simulink model "ddrxpose_21a_generic"  (R2021a)
settings: Solver=VariableStepAuto  StartTime=0.0  StopTime=300e-6  FixedStep=Ts  RelTol=1e-3  EnableMultiTasking=on
InitFcn:
  | model_init_sim;
model workspace (MAT data in the model file):
  mwTaskManagerKernelLatency = 0
  socvcb = containers.Map
  socvcb.serialization.keys = {74.0001220703, 74.0092773438, 74.0178222656, 75.0001220703, 75.0092773438, 75.0178222656}
  socvcb.serialization.values : function handle (value not decoded)
  socvcb.serialization.uniformity = 0
  socvcb.serialization.keyType = 'double'
  socvcb.serialization.valueType = 'any'
values from neighbouring files (symbols this model uses):
  hBlank = 20    [model_init_sim.m]
  inputImageDDROffset = uint32(hex2dec('00000000'))    [model_init_sim.m]
  MatrixInput = reshape(MatrixInputArr,[N1,N2])    [matrix_init.m]
  pAXIDataWidthBytes = 4    [model_init_sim.m]
  pMaxBankLines = 6    [model_init_sim.m]
  pMaxNumBanks = 3    [model_init_sim.m]
  pNumCols = 30    [model_init_sim.m]
  pNumRows = 30    [model_init_sim.m]
  Ts = 1/(totalPixels*60)    [model_init_sim.m]
libraries: socmemlib x2, hdlsllib x2, simulink x1
settings Model: DataTypeOverride=Off  SimulationMode=accelerator  ExtModeTrigDuration=1  Creator=skuznick  LastModifiedBy=darenlee
settings SolverCC: AlgebraicLoopSolver=TrustRegion  PositivePriorityOrder=on
settings DataIOCC: LimitDataPoints=on  SaveOutput=off  DSMLogging=off  InspectSignalLogs=on  VisualizeSimOutput=off  SaveTime=off
settings OptimizationCC: BlockReduction=off  ConditionallyExecuteInputs=off  DefaultUnderspecifiedDataType=single  EnhancedBackFolding=on  PassReuseOutputArgsAs=Individual arguments  ZeroExternalMemoryAtStartup=off  ZeroInternalMemoryAtStartup=off  EfficientFloat2IntCast=on  MaxStackSize=64  SimCompilerOptimization=on  OptimizeBlockOrder=speed  DifferentSizesBufferReuse=on  OptimizationCustomize=off  EfficientTunableParamExpr=on
settings DebuggingCC: AlgebraicLoopMsg=error  SingleTaskRateTransMsg=error  ParameterPrecisionLossMsg=none  ParameterTunabilityLossMsg=error  AllowSymbolicDim=off  PregeneratedLibrarySubsystemCodeDiagnostic=none  SFUnexpectedBacktrackingDiag=warning  SFNoUnconditionalDefaultTransitionDiag=warning  SFExecutionAtInitializationDiag=none  SFMachineParentedDataDiag=warning  IntegerSaturationMsg=none  ArithmeticOperatorsInVariantConditions=warning
settings HardwareCC: ProdBitPerLong=64  ProdLargestAtomicInteger=LongLong  ProdLargestAtomicFloat=Double  ProdLongLongMode=on  ProdHWDeviceType=ARM Compatible->ARM 64-bit (LP64)  ProdEqTarget=off  HardwareBoardFeatureSet=SoCBlockset
settings SFSimCC: SimUseLocalCustomCode=off  MATLABDynamicMemAlloc=off  CustomCodeUndefinedFunction=UseInterfaceOnly
settings RTWCC: SystemTargetFile=ert.tlc  HardwareBoard=Xilinx Zynq UltraScale+ MPSoC ZCU102 Evaluation Kit  TLCOptions="-aInlineSetEventsForThisBaseRateFcn=TLC_FALSE -aSuppressMultiTaskScheduler=TLC_FALSE  -aRateBasedStepFcn=0"  TemplateMakefile=ert_default_tmf  GenerateReport=on  RTWUseLocalCustomCode=off  Toolchain=Linaro AArch64 Linux v6.3.1  BuildConfiguration=Faster Runs  IncludeHyperlinkInReport=on  LaunchReport=on  GenerateTraceInfo=on  GenerateTraceReport=on  GenerateTraceReportSl=on  GenerateTraceReportSf=on  GenerateTraceReportEml=on
settings CodeAppCC: ForceParamTrailComments=on  IgnoreCustomStorageClasses=off  OperatorAnnotations=on  SimulinkDataObjDesc=on  SFDataObjDesc=on  InsertBlockDesc=on
settings ConfigComp: CovMetricSettings=dw  CovSaveCumulativeToWorkspaceVar=on  CovSaveSingleToWorkspaceVar=on  CovExternalEMLEnable=off  CovSFcnEnable=off

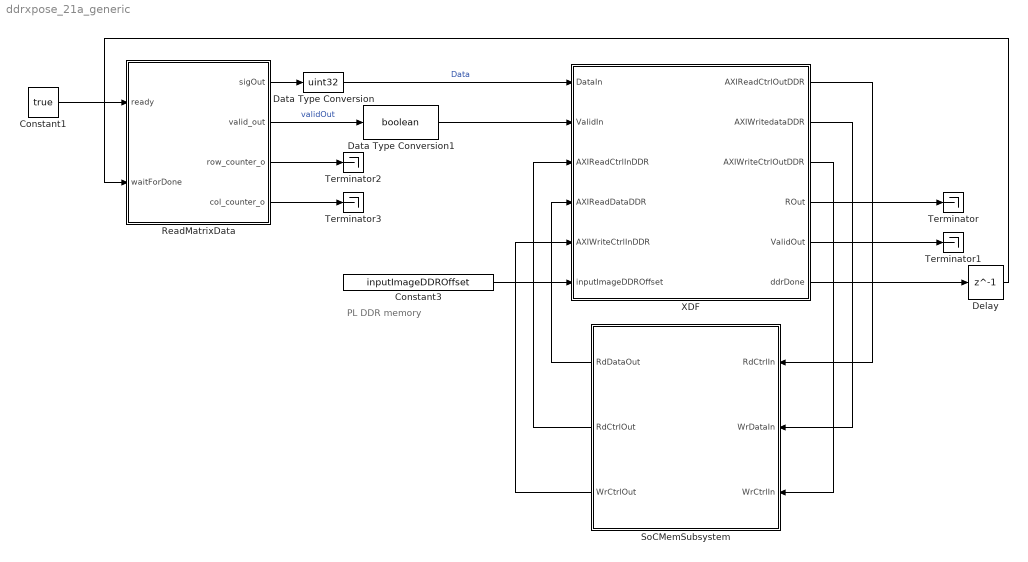
== system ddrxpose_21a_generic ==
  note: PL DDR memory
  Constant1 : Constant  Value=true  SampleTime=-1
  Constant3 : Constant  Value=inputImageDDROffset  OutDataTypeStr=uint32  SampleTime=-1
  Data Type Conversion : DataTypeConversion  OutDataTypeStr=uint32
  Data Type Conversion1 : DataTypeConversion  OutDataTypeStr=boolean
  Delay : Delay  DelayLength=1
  ReadMatrixData : MATLAB Function  TreatAsAtomicUnit=on  SystemSampleTime=Ts  mask{MatrixInput=MatrixInput, ValidGap=16*3 % 48 clock cycles, Ts=Ts}
      mask prompts: MatrixInput "Matrix value"; ValidGap "Valid Gap between columns"; Ts "Sample Time"
  SoCMemSubsystem : Subsystem
  Terminator{,1..3} (4 alike) : Terminator
  XDF : Subsystem  TreatAsAtomicUnit=on
  wires:
  SoCMemSubsystem/2(RdCtrlOut) -> XDF/3(AXIReadCtrlInDDR)
  SoCMemSubsystem/3(WrCtrlOut) -> XDF/5(AXIWriteCtrlInDDR)
  SoCMemSubsystem/1(RdDataOut) -> XDF/4(AXIReadDataDDR)
  XDF/1(AXIReadCtrlOutDDR) -> SoCMemSubsystem/1(RdCtrlIn)
  XDF/2(AXIWritedataDDR) -> SoCMemSubsystem/2(WrDataIn)
  XDF/3(AXIWriteCtrlOutDDR) -> SoCMemSubsystem/3(WrCtrlIn)
  Constant3/1 -> XDF/6(inputImageDDROffset)
  XDF/6(ddrDone) -> Delay/1
  Constant1/1 -> ReadMatrixData/1(ready)
  ReadMatrixData/1(sigOut) -> Data Type Conversion/1
  ReadMatrixData/2(valid_out) -> Data Type Conversion1/1  "validOut"
  ReadMatrixData/3(row_counter_o) -> Terminator2/1
  ReadMatrixData/4(col_counter_o) -> Terminator3/1
  Data Type Conversion/1 -> XDF/1(DataIn)  "Data"
  Delay/1 -> ReadMatrixData/2(waitForDone)
  XDF/4(ROut) -> Terminator/1
  XDF/5(ValidOut) -> Terminator1/1
  Data Type Conversion1/1 -> XDF/2(ValidIn)

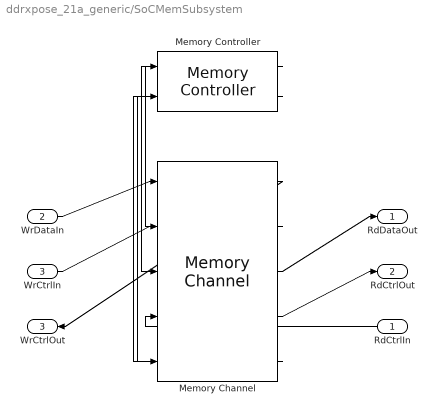
== system ddrxpose_21a_generic/SoCMemSubsystem ==
  RdCtrlIn : Inport
  WrDataIn : Inport  Port=2
  WrCtrlIn : Inport  Port=3
  Memory Channel : socmemlib/Memory Channel  InstantiateOnLoad=on  ChannelType=AXI4 Random Access  MRBufferSize=pNumCols*pNumRows*4*4  MRNumBuffers=1  BurstLengthWriterChIf=256  BurstLengthReaderChIf=256  UseValuesFromTargetHardwareResources=off  ReaderWriterUseSameValues=on  FIFODepthWriter=8  FIFODepthReader=8  FIFOAFullDepthWriter=6  FIFOAFullDepthReader=6  ICClockFrequencyWriter=300  ICClockFrequencyReader=300  ICDataWidthWriter=32  ICDataWidthReader=32  ChDimensionsWriterChIf=1  ChTypeWriterChIf=fixdt(0,(pAXIDataWidthBytes*8),0)  ChFrameSampleTimeWriterChIf=Ts  ChBitPackedWriterChIf=off  OutSigSpecMatchesInSigSpec=on  ChDimensionsReaderChIf=1  ChTypeWithInhReaderChIf=uint8  ChFrameSampleTimeReaderChIf=6.734006734006734e-09  ChBitPackedReaderChIf=off  InsertInactivePixelClocksReaderChIf=off  FrameSizeReaderChIf=160x120p  ProtocolWriter=AXI4  ProtocolReader=AXI4  ChTypeReaderChIf=fixdt(0,32,0)  LastTargetBoard=Xilinx Zynq UltraScale+ MPSoC ZCU102 Evaluation Kit  Beta2Compatible=off  MRRegionSize=14400  DiagnosticLevel=Basic diagnostic signals  MRBaseAddress=hex2dec('00010000')  UseTargetGlobalValues=off  InterruptHandlingTimeWriterChIf=10e-6  BufferEventIDWriterChIf=NOT_USED  BufferLengthReaderChIf=NOT_USED  InterruptHandlingTimeReaderChIf=10e-6  BufferEventIDReaderChIf=NOT_USED
      settings: SourceProductBaseCode=HW
  Memory Controller : socmemlib/Memory Controller  InstantiateOnLoad=on  NumMasters=2  ICArbitrationPolicy=Round robin  UseValuesFromTargetHardwareResources=off  ControllerFrequency=300  ControllerDataWidth=128  BandwidthDerating=2.3  WriteFirstTransferLatency=19  ReadFirstTransferLatency=2  WriteLastTransferLatency=4  ReadLastTransferLatency=1  LastTargetBoard=Xilinx Zynq UltraScale+ MPSoC ZCU102 Evaluation Kit  DiagnosticLevel=Basic diagnostic signals.2  MAX_NUM_MASTERS=12  DDRRefreshLength=4  DDRRefreshInterval=7.8  PlotTimeResolution=100e-6
      settings: SourceProductBaseCode=HW
  RdDataOut : Outport  VectorParamsAs1DForOutWhenUnconnected=off
  RdCtrlOut : Outport  Port=2  VectorParamsAs1DForOutWhenUnconnected=off
  WrCtrlOut : Outport  Port=3  VectorParamsAs1DForOutWhenUnconnected=off
  wires:
  Memory Channel/3 -> RdDataOut/1
  Memory Channel/4 -> RdCtrlOut/1
  Memory Channel/1 -> WrCtrlOut/1
  RdCtrlIn/1 -> Memory Channel/4
  WrDataIn/1 -> Memory Channel/1
  WrCtrlIn/1 -> Memory Channel/2
  Memory Channel/2 -> Memory Controller/1
  Memory Controller/1 -> Memory Channel/3
  Memory Controller/2 -> Memory Channel/5
  Memory Channel/5 -> Memory Controller/2

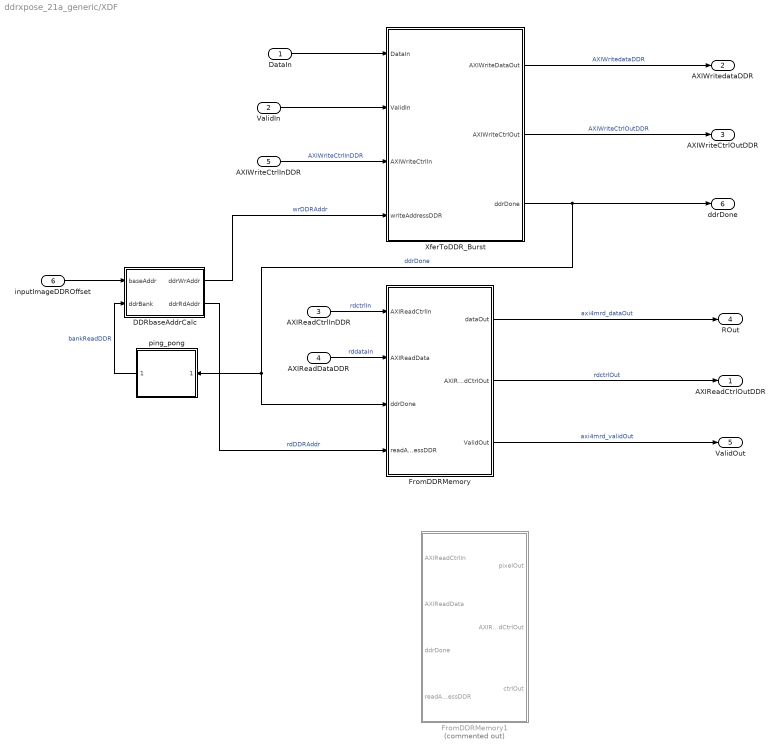
== system ddrxpose_21a_generic/XDF ==
  DataIn : Inport
  ValidIn : Inport  Port=2
  AXIReadCtrlInDDR : Inport  Port=3
  AXIReadDataDDR : Inport  Port=4
  AXIWriteCtrlInDDR : Inport  Port=5
  inputImageDDROffset : Inport  Port=6
  DDRbaseAddrCalc : Subsystem
  FromDDRMemory : Subsystem
  FromDDRMemory1 : Subsystem  Commented=on
  XferToDDR_Burst : Subsystem  VariantControl=XferToDDR_Burst
  ping_pong : Subsystem
  AXIReadCtrlOutDDR : Outport  VectorParamsAs1DForOutWhenUnconnected=off
  AXIWritedataDDR : Outport  Port=2  VectorParamsAs1DForOutWhenUnconnected=off
  AXIWriteCtrlOutDDR : Outport  Port=3  VectorParamsAs1DForOutWhenUnconnected=off
  ROut : Outport  Port=4  VectorParamsAs1DForOutWhenUnconnected=off
  ValidOut : Outport  Port=5
  ddrDone : Outport  Port=6
  wires:
  AXIWriteCtrlInDDR/1 -> XferToDDR_Burst/3(AXIWriteCtrlIn)  "AXIWriteCtrlInDDR"
  XferToDDR_Burst/1(AXIWriteDataOut) -> AXIWritedataDDR/1  "AXIWritedataDDR"
  XferToDDR_Burst/2(AXIWriteCtrlOut) -> AXIWriteCtrlOutDDR/1  "AXIWriteCtrlOutDDR"
  AXIReadCtrlInDDR/1 -> FromDDRMemory/1(AXIReadCtrlIn)  "rdctrlIn"
  AXIReadDataDDR/1 -> FromDDRMemory/2(AXIReadData)  "rddataIn"
  XferToDDR_Burst/3(ddrDone) -> ping_pong/1(ddrDone), FromDDRMemory/3(ddrDone), ddrDone/1  "ddrDone"
  FromDDRMemory/1(dataOut) -> ROut/1  "axi4mrd_dataOut"
  FromDDRMemory/2(AXIReadCtrlOut) -> AXIReadCtrlOutDDR/1  "rdctrlOut"
  DDRbaseAddrCalc/1(ddrWrAddr) -> XferToDDR_Burst/4(writeAddressDDR)  "wrDDRAddr"
  inputImageDDROffset/1 -> DDRbaseAddrCalc/1(baseAddr)
  ping_pong/1(ddrBank) -> DDRbaseAddrCalc/2(ddrBank)  "bankReadDDR"
  DDRbaseAddrCalc/2(ddrRdAddr) -> FromDDRMemory/4(readAddressDDR)  "rdDDRAddr"
  DataIn/1 -> XferToDDR_Burst/1(DataIn)
  ValidIn/1 -> XferToDDR_Burst/2(ValidIn)
  FromDDRMemory/3(ValidOut) -> ValidOut/1  "axi4mrd_validOut"

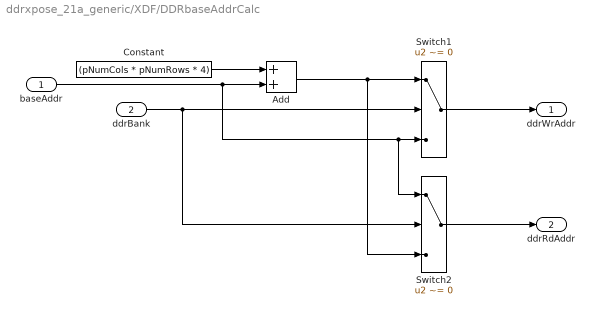
== system ddrxpose_21a_generic/XDF/DDRbaseAddrCalc ==
  baseAddr : Inport
  ddrBank : Inport  Port=2
  Add : Sum  OutDataTypeStr=uint32
  Constant : Constant  Value=(pNumCols * pNumRows * 4)  OutDataTypeStr=uint32  SampleTime=-1
  Switch1 : Switch  Criteria=u2 ~= 0
  Switch2 : Switch  Criteria=u2 ~= 0
  ddrWrAddr : Outport
  ddrRdAddr : Outport  Port=2
  wires:
  Constant/1 -> Add/1
  Add/1 -> Switch2/3, Switch1/1
  Switch1/1 -> ddrWrAddr/1
  ddrBank/1 -> Switch2/2, Switch1/2
  baseAddr/1 -> Switch2/1, Switch1/3, Add/2
  Switch2/1 -> ddrRdAddr/1

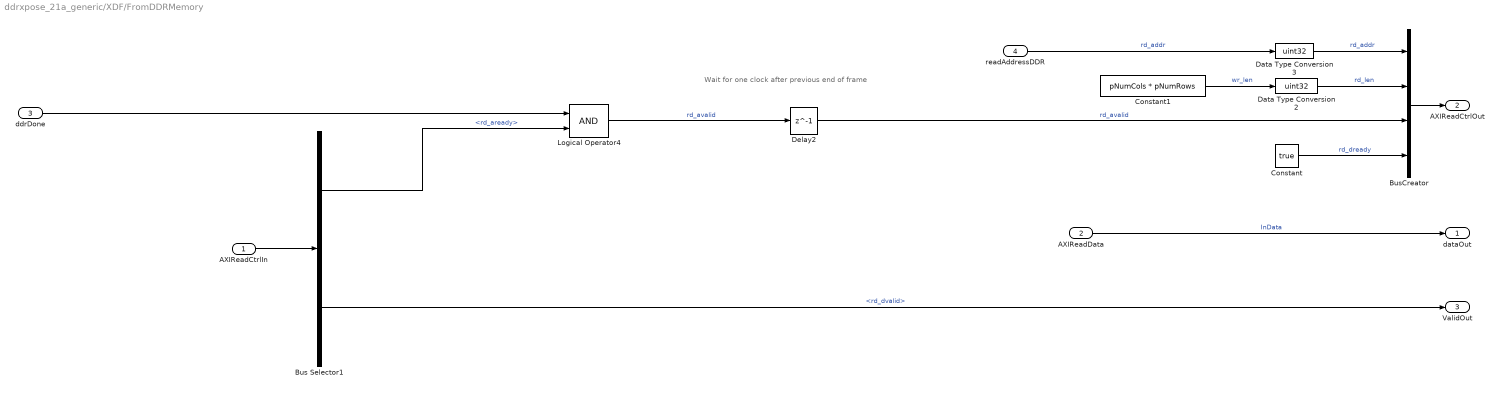
== system ddrxpose_21a_generic/XDF/FromDDRMemory ==
  note: Wait for one clock after previous end of frame
  AXIReadCtrlIn : Inport
  AXIReadData : Inport  Port=2
  ddrDone : Inport  Port=3
  readAddressDDR : Inport  Port=4
  Bus Selector1 : BusSelector  OutputSignals=rd_aready,rd_dvalid
  BusCreator : BusCreator  Inputs=4
  Constant : Constant  Value=true  SampleTime=-1
  Constant1 : Constant  Value=pNumCols * pNumRows  OutDataTypeStr=uint32  SampleTime=-1
  Data Type Conversion2 : DataTypeConversion  OutDataTypeStr=uint32
  Data Type Conversion3 : DataTypeConversion  OutDataTypeStr=uint32
  Delay2 : Delay  DelayLength=1  InitialCondition=0
  Logical Operator4 : Logic  IconShape=distinctive  AllPortsSameDT=off  OutDataTypeStr=boolean
  dataOut : Outport  VectorParamsAs1DForOutWhenUnconnected=off
  AXIReadCtrlOut : Outport  Port=2  VectorParamsAs1DForOutWhenUnconnected=off
  ValidOut : Outport  Port=3
  wires:
  Delay2/1 -> BusCreator/3  "rd_avalid"
  Constant/1 -> BusCreator/4  "rd_dready"
  Bus Selector1/1 -> Logical Operator4/2  "<rd_aready>"
  BusCreator/1 -> AXIReadCtrlOut/1
  Bus Selector1/2 -> ValidOut/1  "<rd_dvalid>"
  Logical Operator4/1 -> Delay2/1  "rd_avalid"
  AXIReadData/1 -> dataOut/1  "InData"
  Constant1/1 -> Data Type Conversion2/1  "wr_len"
  Data Type Conversion2/1 -> BusCreator/2  "rd_len"
  AXIReadCtrlIn/1 -> Bus Selector1/1
  Data Type Conversion3/1 -> BusCreator/1  "rd_addr"
  readAddressDDR/1 -> Data Type Conversion3/1  "rd_addr"
  ddrDone/1 -> Logical Operator4/1

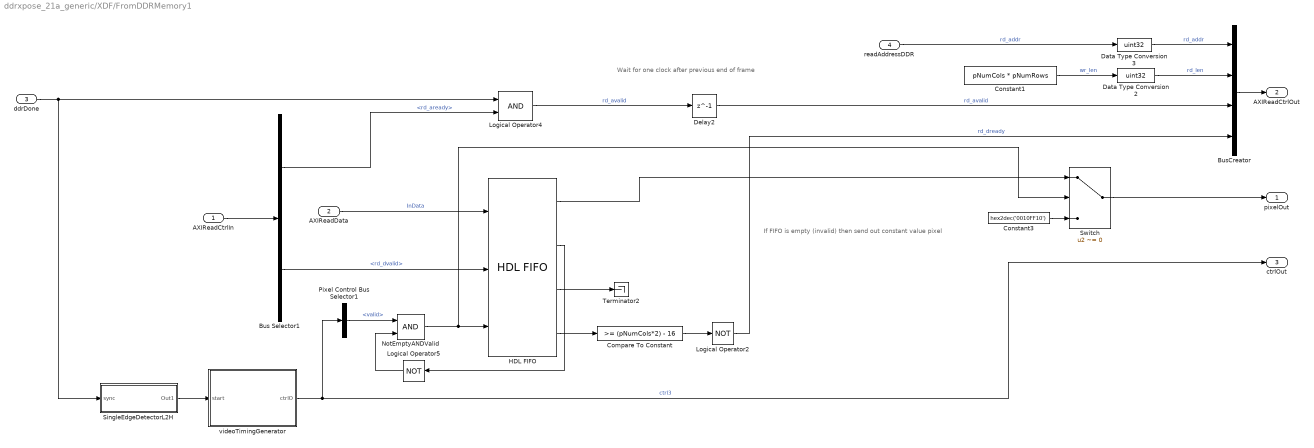
== system ddrxpose_21a_generic/XDF/FromDDRMemory1 ==
  note: Wait for one clock after previous end of frame
  note: If FIFO is empty (invalid) then send out constant value pixel
  AXIReadCtrlIn : Inport
  AXIReadData : Inport  Port=2
  ddrDone : Inport  Port=3
  readAddressDDR : Inport  Port=4
  Bus Selector1 : BusSelector  OutputSignals=rd_aready,rd_dvalid
  BusCreator : BusCreator  Inputs=4
  Compare To Constant : simulink/Logic and Bit Operations/Compare To Constant  relop=>=  const=(pNumCols*2) - 16  OutDataTypeStr=boolean
  Constant1 : Constant  Value=pNumCols * pNumRows  OutDataTypeStr=uint32  SampleTime=-1
  Constant3 : Constant  Value=hex2dec('0010FF10')  OutDataTypeStr=fixdt(0,32,0)  SampleTime=-1
  Data Type Conversion2 : DataTypeConversion  OutDataTypeStr=uint32
  Data Type Conversion3 : DataTypeConversion  OutDataTypeStr=uint32
  Delay2 : Delay  DelayLength=1  InitialCondition=0
  HDL FIFO : hdlsllib/HDL RAMs/HDL FIFO  fifo_size=pNumCols*2  mode=FWFT  ratio=1  push_msg=Warning  pop_msg=Warning  show_empty=on  show_full=on  show_num=on  LabelModeActiveChoice_Mode=FWFT
      settings: SourceProductBaseCode=SL
  Logical Operator2 : Logic  Operator=NOT  IconShape=distinctive  AllPortsSameDT=off  OutDataTypeStr=boolean
  Logical Operator4 : Logic  IconShape=distinctive  AllPortsSameDT=off  OutDataTypeStr=boolean
  Logical Operator5 : Logic  Operator=NOT  IconShape=distinctive  AllPortsSameDT=off  OutDataTypeStr=boolean
  NotEmptyANDValid : Logic  IconShape=distinctive  AllPortsSameDT=off  OutDataTypeStr=boolean
  Pixel Control Bus Selector1 : BusSelector  OutputSignals=valid
  SingleEdgeDetectorL2H : Subsystem  TreatAsAtomicUnit=on
  Switch : Switch  Criteria=u2 ~= 0
  Terminator2 : Terminator
  videoTimingGenerator : MATLAB Function  TreatAsAtomicUnit=on  VariantControl=Variant2  mask{hSize=pNumCols, vSize=pNumRows, hBlank=hBlank, vBlank=2, delayStartClks=pNumCols*5}
      mask prompts: hSize "Frame Width"; vSize "Frame Height"; hBlank "Horz Blanking"; vBlank "Vert Blanking"; delayStartClks "Start Delay in Clocks"
  pixelOut : Outport  VectorParamsAs1DForOutWhenUnconnected=off
  AXIReadCtrlOut : Outport  Port=2  VectorParamsAs1DForOutWhenUnconnected=off
  ctrlOut : Outport  Port=3  VectorParamsAs1DForOutWhenUnconnected=off
  wires:
  Switch/1 -> pixelOut/1
  NotEmptyANDValid/1 -> Switch/2, HDL FIFO/3
  Constant3/1 -> Switch/3
  Delay2/1 -> BusCreator/3  "rd_avalid"
  Logical Operator2/1 -> BusCreator/4  "rd_dready"
  Pixel Control Bus Selector1/1 -> NotEmptyANDValid/1  "<valid>"
  HDL FIFO/1 -> Switch/1
  Bus Selector1/1 -> Logical Operator4/2  "<rd_aready>"
  Logical Operator5/1 -> NotEmptyANDValid/2
  BusCreator/1 -> AXIReadCtrlOut/1
  Bus Selector1/2 -> HDL FIFO/2  "<rd_dvalid>"
  Logical Operator4/1 -> Delay2/1  "rd_avalid"
  HDL FIFO/2 -> Logical Operator5/1
  AXIReadData/1 -> HDL FIFO/1  "InData"
  Constant1/1 -> Data Type Conversion2/1  "wr_len"
  Data Type Conversion2/1 -> BusCreator/2  "rd_len"
  AXIReadCtrlIn/1 -> Bus Selector1/1
  Data Type Conversion3/1 -> BusCreator/1  "rd_addr"
  readAddressDDR/1 -> Data Type Conversion3/1  "rd_addr"
  HDL FIFO/4 -> Compare To Constant/1
  Compare To Constant/1 -> Logical Operator2/1
  HDL FIFO/3 -> Terminator2/1
  videoTimingGenerator/1(ctrlO) -> ctrlOut/1, Pixel Control Bus Selector1/1  "ctrl3"
  ddrDone/1 -> SingleEdgeDetectorL2H/1(sync), Logical Operator4/1
  SingleEdgeDetectorL2H/1(Out1) -> videoTimingGenerator/1(start)

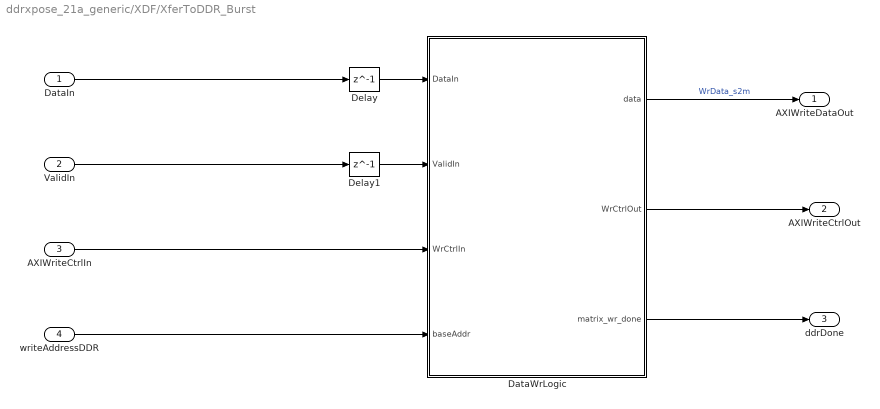
== system ddrxpose_21a_generic/XDF/XferToDDR_Burst ==
  DataIn : Inport
  ValidIn : Inport  Port=2
  AXIWriteCtrlIn : Inport  Port=3
  writeAddressDDR : Inport  Port=4
  DataWrLogic : Subsystem
  Delay : Delay  DelayLength=1
  Delay1 : Delay  DelayLength=1
  AXIWriteDataOut : Outport
  AXIWriteCtrlOut : Outport  Port=2
  ddrDone : Outport  Port=3
  wires:
  Delay1/1 -> DataWrLogic/2(ValidIn)
  Delay/1 -> DataWrLogic/1(DataIn)
  DataWrLogic/1(data) -> AXIWriteDataOut/1  "WrData_s2m"
  DataIn/1 -> Delay/1
  DataWrLogic/2(WrCtrlOut) -> AXIWriteCtrlOut/1
  AXIWriteCtrlIn/1 -> DataWrLogic/3(WrCtrlIn)
  DataWrLogic/3(matrix_wr_done) -> ddrDone/1
  ValidIn/1 -> Delay1/1
  writeAddressDDR/1 -> DataWrLogic/4(baseAddr)

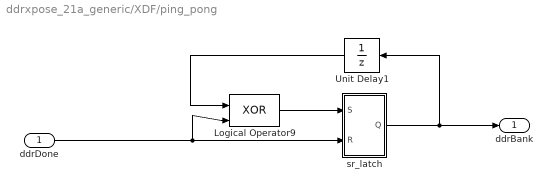
== system ddrxpose_21a_generic/XDF/ping_pong ==
  ddrDone : Inport
  Logical Operator9 : Logic  Operator=XOR  IconShape=distinctive  AllPortsSameDT=off  OutDataTypeStr=boolean
  Unit Delay1 : UnitDelay  SampleTime=-1  HasFrameUpgradeWarning=on
  sr_latch : Subsystem
  ddrBank : Outport  VectorParamsAs1DForOutWhenUnconnected=off
  wires:
  Unit Delay1/1 -> Logical Operator9/1
  Logical Operator9/1 -> sr_latch/1(S)
  ddrDone/1 -> sr_latch/2(R), Logical Operator9/2
  sr_latch/1(Q) -> Unit Delay1/1, ddrBank/1

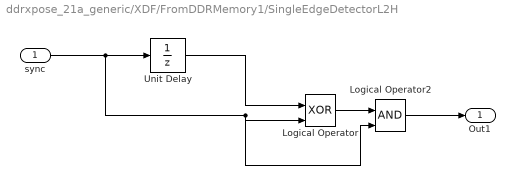
== system ddrxpose_21a_generic/XDF/FromDDRMemory1/SingleEdgeDetectorL2H ==
  sync : Inport  OutDataTypeStr=boolean
  Logical Operator : Logic  Operator=XOR  IconShape=distinctive  AllPortsSameDT=off  OutDataTypeStr=boolean
  Logical Operator2 : Logic  IconShape=distinctive  AllPortsSameDT=off  OutDataTypeStr=boolean
  Unit Delay : UnitDelay  SampleTime=-1  HasFrameUpgradeWarning=on
  Out1 : Outport  VectorParamsAs1DForOutWhenUnconnected=off
  wires:
  Logical Operator2/1 -> Out1/1
  Logical Operator/1 -> Logical Operator2/1
  Unit Delay/1 -> Logical Operator/1
  sync/1 -> Logical Operator2/2, Logical Operator/2, Unit Delay/1

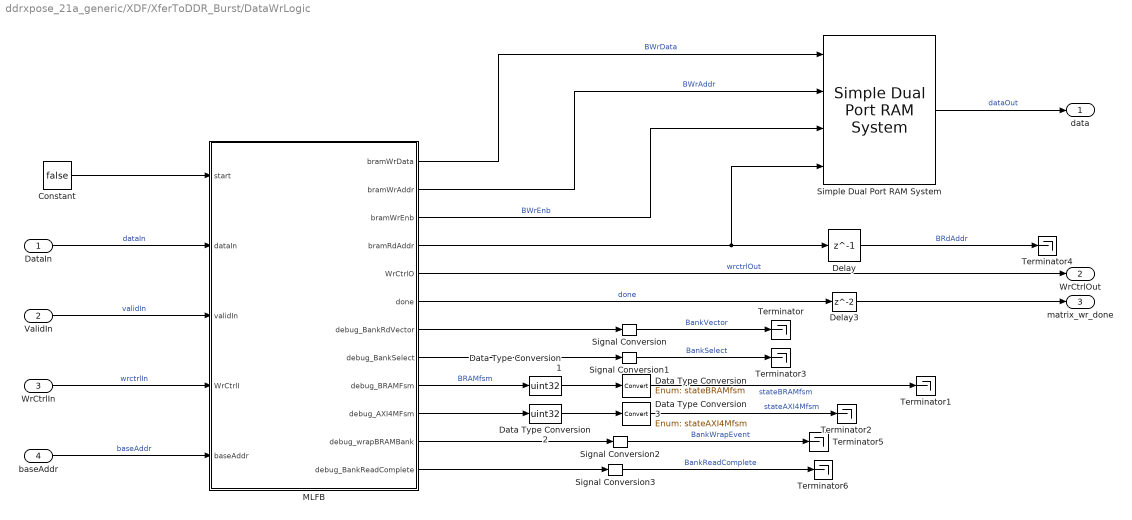
== system ddrxpose_21a_generic/XDF/XferToDDR_Burst/DataWrLogic ==
  DataIn : Inport
  ValidIn : Inport  Port=2
  WrCtrlIn : Inport  Port=3
  baseAddr : Inport  Port=4
  Constant : Constant  Value=false  SampleTime=-1
  Data Type Conversion : DataTypeConversion  OutDataTypeStr=Enum: stateBRAMfsm
  Data Type Conversion1 : DataTypeConversion  OutDataTypeStr=uint32
  Data Type Conversion2 : DataTypeConversion  OutDataTypeStr=uint32
  Data Type Conversion3 : DataTypeConversion  OutDataTypeStr=Enum: stateAXI4Mfsm
  Delay : Delay  DelayLength=1
  Delay3 : Delay
  MLFB : MATLAB Function  TreatAsAtomicUnit=on
  Signal Conversion{,1..3} (4 alike) : SignalConversion  OverrideOpt=off
  Simple Dual Port RAM System : hdlsllib/HDL RAMs/Simple Dual Port RAM System  RAMType=Simple dual port  WriteOutputValue=New data  RAMInitialValue=0  SimulateUsing=Code generation
      settings: SourceProductBaseCode=SL
  Terminator{,1..6} (7 alike) : Terminator
  data : Outport
  WrCtrlOut : Outport  Port=2
  matrix_wr_done : Outport  Port=3
  wires:
  MLFB/6(done) -> Delay3/1  "done"
  MLFB/5(WrCtrlO) -> WrCtrlOut/1  "wrctrlOut"
  Simple Dual Port RAM System/1 -> data/1  "dataOut"
  baseAddr/1 -> MLFB/5(baseAddr)  "baseAddr"
  WrCtrlIn/1 -> MLFB/4(WrCtrlI)  "wrctrlIn"
  MLFB/1(bramWrData) -> Simple Dual Port RAM System/1  "BWrData"
  ValidIn/1 -> MLFB/3(validIn)  "validIn"
  DataIn/1 -> MLFB/2(dataIn)  "dataIn"
  MLFB/4(bramRdAddr) -> Simple Dual Port RAM System/4, Delay/1
  MLFB/2(bramWrAddr) -> Simple Dual Port RAM System/2  "BWrAddr"
  MLFB/3(bramWrEnb) -> Simple Dual Port RAM System/3  "BWrEnb"
  Delay3/1 -> matrix_wr_done/1
  MLFB/7(debug_BankRdVector) -> Signal Conversion/1
  MLFB/9(debug_BRAMFsm) -> Data Type Conversion1/1  "BRAMfsm"
  MLFB/10(debug_AXI4MFsm) -> Data Type Conversion2/1
  Data Type Conversion/1 -> Terminator1/1  "stateBRAMfsm"
  Data Type Conversion1/1 -> Data Type Conversion/1
  Data Type Conversion2/1 -> Data Type Conversion3/1
  Data Type Conversion3/1 -> Terminator2/1  "stateAXI4Mfsm"
  Signal Conversion/1 -> Terminator/1  "BankVector"
  MLFB/8(debug_BankSelect) -> Signal Conversion1/1
  Signal Conversion1/1 -> Terminator3/1  "BankSelect"
  Delay/1 -> Terminator4/1  "BRdAddr"
  MLFB/11(debug_wrapBRAMBank) -> Signal Conversion2/1
  Signal Conversion2/1 -> Terminator5/1  "BankWrapEvent"
  MLFB/12(debug_BankReadComplete) -> Signal Conversion3/1
  Signal Conversion3/1 -> Terminator6/1  "BankReadComplete"
  Constant/1 -> MLFB/1(start)

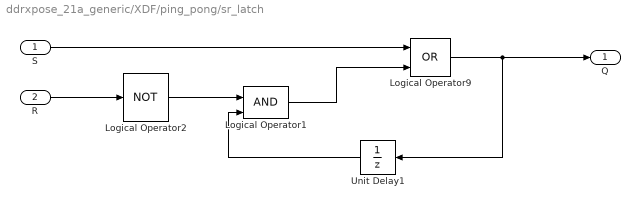
== system ddrxpose_21a_generic/XDF/ping_pong/sr_latch ==
  S : Inport
  R : Inport  Port=2
  Logical Operator1 : Logic  IconShape=distinctive  AllPortsSameDT=off  OutDataTypeStr=boolean
  Logical Operator2 : Logic  Operator=NOT  IconShape=distinctive  AllPortsSameDT=off  OutDataTypeStr=boolean
  Logical Operator9 : Logic  Operator=OR  IconShape=distinctive  AllPortsSameDT=off  OutDataTypeStr=boolean
  Unit Delay1 : UnitDelay  SampleTime=-1  HasFrameUpgradeWarning=on
  Q : Outport  VectorParamsAs1DForOutWhenUnconnected=off
  wires:
  Logical Operator9/1 -> Q/1, Unit Delay1/1
  Unit Delay1/1 -> Logical Operator1/2
  S/1 -> Logical Operator9/1
  R/1 -> Logical Operator2/1
  Logical Operator2/1 -> Logical Operator1/1
  Logical Operator1/1 -> Logical Operator9/2

== matlab function ddrxpose_21a_generic/XDF/XferToDDR_Burst/DataWrLogic/MLFB ==
  data: bramWrData output; bramWrAddr output; bramWrEnb output; bramRdAddr output; WrCtrlO output Bus: WriteControlM2SBusObj; done output; start input; dataIn input; validIn input; WrCtrlI input; baseAddr input; debug_BankRdVector output; debug_BankSelect output; debug_BRAMFsm output; pNumCols parameter; pNumRows parameter; pMaxBankLines parameter; pMaxNumBanks parameter; pAXIDataWidthBytes parameter; debug_AXI4MFsm output; debug_wrapBRAMBank output; debug_BankReadComplete output
function [bramWrData, bramWrAddr, bramWrEnb, bramRdAddr, WrCtrlO, done, debug_BankRdVector, debug_BankSelect, debug_BRAMFsm, debug_AXI4MFsm, debug_wrapBRAMBank, debug_BankReadComplete] =  ...
burstTranspose(start, dataIn, validIn, WrCtrlI, baseAddr, pNumCols, pNumRows, pMaxBankLines, pMaxNumBanks, pAXIDataWidthBytes)

% define FSM States
IDLE = fi(0,0,4,0);
% States for managing the writing to BRAM
LINEBUFFER = fi(1,0,4,0);
LINESTART = fi(3,0,4,0);
% States for managing the writing to DDR
BURSTSTART = fi(1,0,4,0);
BURSTNEXT  = fi(3,0,4,0);
WAITBURSTCOMPLETE = fi(4,0,4,0);
WAITBURSTREADY = fi(5,0,4,0);
WAITONBANKRDY =fi(2,0,4,0);

% pAXIDataWidthBytes = coder.const(16);
% maxBufLines = uint16(4);

persistent stateBRAMfsm burstState WrBank RdBank WrData BankRdy WrAddr RdAddr WrEnb colCnt rowCnt WrBankLine RdBankLine WrDone aximWrAddr aximWrValid startRdAddr burstCount aximWrLen aximNumRowsWritten bankWrWrap
if isempty(stateBRAMfsm)
    stateBRAMfsm = IDLE;
    burstState = IDLE;
    bankWrWrap = false;
    WrBank = fi(0,0,8,0);
    RdBank = fi(0,0,8,0);
    BankRdy = zeros(uint32(pMaxNumBanks),1,'logical');
    WrBankLine = uint16(0);
    RdBankLine = uint16(0);
    WrEnb = false;
    WrDone = false;
    aximWrAddr = uint32(0);
    aximWrLen = uint32(pMaxBankLines);
    aximWrValid = false;
    WrData = cast(0,'like', dataIn);
%     WrAddr = fi(0,0,14,0);
%     RdAddr = fi(0,0,14,0);
    WrAddr = fi(0,0,10,0);
    RdAddr = cast(0,'like',WrAddr);
    startRdAddr = cast(0,'like',WrAddr);
    burstCount = uint16(0);
    colCnt = fi(0,0,ceil(log2(pNumCols)),0);
    rowCnt = fi(0,0,ceil(log2(pNumRows)),0);
    aximNumRowsWritten = uint32(0);
end

bramWrData = WrData;
bramWrEnb = WrEnb;
bramWrAddr = WrAddr;
bramRdAddr = RdAddr;
wr_ddr_addr = uint32((aximWrAddr * pAXIDataWidthBytes) + baseAddr);
WrCtrlO = struct('wr_addr', wr_ddr_addr, 'wr_len', aximWrLen, 'wr_valid', aximWrValid);
done = WrDone;
WrDone = false;  % Note: WrDone true for one clock only

% if aximWrValid
%     fprintf("+DDR: RdAddr@ %u RdBankLine %u RdBank %u AXIMAddr: %u AXIMLen: %u\n", uint32(RdAddr), RdBankLine, uint16(RdBank), aximWrAddr, aximWrLen);
% end


%% For debug outputs only
debug_BankRdVector = BankRdy; % display status of each BRAM bank. if a 1 is written to a bank, it means it  has data that has NOT been fully read out yet
debug_BankSelect = WrBank;  % which BRAM bank is selected to write new data to. Zero indexed
debug_wrapBRAMBank = bankWrWrap; % Will occur when we wrap to the first BRAM Bank
debug_BankReadComplete = (RdBankLine == 0); % finished reading a bank (got to end of column) and reset to zero event

debug_BRAMFsm = stateBRAMfsm; % BRAM write state machine
debug_AXI4MFsm = burstState;  % BRAM Read -> DDR4 state machine



%%

% process col and row counts
if WrEnb  % write to BRAM
%     fprintf("+BRAM: %08x @ %u Col %u Row %u WrBankLine %u WrBank %u\n", uint32(WrData), uint32(WrAddr), uint16(colCnt), uint16(rowCnt), WrBankLine, uint16(WrBank));
    if colCnt == pNumCols-1
        if rowCnt == pNumRows-1 % end of matrix
            BankRdy(WrBank+1) = true;
            WrBank(:) = WrBank + 1;
            if WrBank == pMaxNumBanks
                WrBank(:) = 0;
                WrAddr(:) = 0;
            end
            stateBRAMfsm = IDLE;
        else
            colCnt(:) = 0;
            rowCnt(:) = rowCnt + 1;
            WrBankLine(:) = WrBankLine + 1;
            if WrBankLine == pMaxBankLines
                BankRdy(WrBank+1) = true;
                if burstState == IDLE
                    burstState = BURSTSTART;
                    startRdAddr(:) = 0;
                end
                WrBankLine(:) = 0;
                WrBank(:) = WrBank + 1;
                % NOTE wrap around to bank 0 
                % The Number of banks might need to change to keep up with
                % the write to DDR rate - keep track of possible collision
                if WrBank == pMaxNumBanks
                    bankWrWrap = true;
                    WrBank(:) = 0;
                    WrAddr(:) = 0;
                end
                if  BankRdy(WrBank+1) == true
                    error('Bank Overrun! Increase number of available banks in BRAM.');
                end
                % WrAddr(:) = WrBank * (numCols*maxBufLines);
            end
        end
    else
        colCnt(:) = colCnt + 1;
    end
end

% reset these after every write
WrEnb = false;

% FSM to manage writing input data to BRAM
switch stateBRAMfsm
    case IDLE
        % first validIn could be on a later clock or on this clock
        if validIn
            WrAddr(:) = 0;
            colCnt(:) = 0;
            rowCnt(:) = 0;
            WrBank(:) = 0;
            BankRdy = zeros(uint32(pMaxNumBanks),1,'logical');
            WrBankLine(:) = 0;
            RdBank(:) = 0;
            
            WrData = dataIn;
            WrEnb = true;
            stateBRAMfsm = LINEBUFFER;
        end
    case LINESTART
        if validIn
            WrData = dataIn;
            WrEnb = true; 
            stateBRAMfsm = LINEBUFFER;
        end
    case LINEBUFFER
        if validIn
            if bankWrWrap
                WrAddr(:) = 0;
                bankWrWrap = false;
            else
                WrAddr(:) = WrAddr + 1;
            end
            WrData = dataIn;
            WrEnb = true; 
        end
end

% FSM To manage the Write to DDR in Bursts in maxBufLines
switch burstState
    case IDLE
    case BURSTSTART
        aximWrAddr(:) = 0; % (bank-1) * maxBufLines;
        RdAddr = startRdAddr ;
        burstCount(:) = 0;
        if BankRdy(RdBank+1) == true
            burstState = WAITBURSTREADY;
        else
            burstState = WAITONBANKRDY;
        end
    case WAITBURSTREADY
        if WrCtrlI.wr_ready
            aximWrValid = true;
            RdAddr(:) = RdAddr + pNumCols;
            burstState(:) = BURSTNEXT;
            burstCount(:) = burstCount + 1;
            if burstCount == aximWrLen
                burstState = WAITBURSTCOMPLETE;
                burstCount(:) = 0;
            end
        else
           aximWrValid = false;
        end
    case BURSTNEXT
        if WrCtrlI.wr_ready
            aximWrValid = true;
            RdAddr(:) = RdAddr + pNumCols;
            burstCount(:) = burstCount + 1;
            if burstCount == aximWrLen
                burstState = WAITBURSTCOMPLETE;
                burstCount(:) = 0;
            end
        else
            aximWrValid = false;
            burstState = WAITBURSTREADY;
        end
    case WAITBURSTCOMPLETE
        aximWrValid = false;
        if WrCtrlI.wr_complete
%          if WrCtrlI.wr_ready  % support pipelined writes (R2020a+)
            aximWrAddr(:) = aximWrAddr + pNumRows;
            % go to next burst of maxBufLines
            startRdAddr(:) = startRdAddr + 1; 
            burstState = WAITBURSTREADY;
            RdBankLine(:) = RdBankLine + 1;
            if RdBankLine == pNumCols   % Reached the end of a bank, need to move to next bank
                RdBankLine(:) = 0;
                BankRdy(RdBank+1) = false;
                RdBank(:) = RdBank + 1;
                if RdBank == pMaxNumBanks
                    RdBank(:) = 0;
                    startRdAddr(:) = 0;
                end
                startRdAddr(:) = uint16(RdBank) * coder.const((pNumCols * pMaxBankLines));  
                aximNumRowsWritten(:) = aximNumRowsWritten + aximWrLen;
                if (pNumRows - aximNumRowsWritten) < pMaxBankLines
                    aximWrLen(:) = pNumRows - aximNumRowsWritten;
                end
                aximWrAddr(:) = aximNumRowsWritten;
                if BankRdy(RdBank+1) == false
                    burstState = WAITONBANKRDY;
%                     fprintf('WAITING for Ready Bank: %u\n', uint32(RdBank));
                end
                if aximNumRowsWritten == pNumRows
                    aximWrLen = uint32(pMaxBankLines);
                    aximNumRowsWritten(:)  = 0;
                    burstState(:) = IDLE;
                    WrDone = true;
                end
            end
            RdAddr(:) = startRdAddr; 
        end        
    case WAITONBANKRDY
        if BankRdy(RdBank+1) == true
            burstState = WAITBURSTREADY;
        end
end

== matlab function ddrxpose_21a_generic/ReadMatrixData ==
  data: sigOut output; valid_out output; MatrixInput parameter; row_counter_o output; col_counter_o output; ValidGap parameter; ready input; waitForDone input
function [sigOut,valid_out,row_counter_o,col_counter_o] = fcn(MatrixInput,ValidGap, ready, waitForDone)
    persistent row_counter col_counter stop_write;
%     ValidGap = 10;
    if isempty(row_counter)
        row_counter = uint32(1);
        col_counter = uint32(1);
        stop_write = false;
      
    end
    [n_rows,m_cols] = size(MatrixInput);
    max_row_count = n_rows + ValidGap;

    %% Read value from matrix
    if row_counter <= n_rows && ~stop_write
        sigOut = MatrixInput(row_counter,col_counter);
        valid_out = true;
    else
        sigOut = 0; % insert valid gap 
        valid_out = false;
    end
    
    row_counter_o = row_counter;
    col_counter_o = col_counter;
    
    %% Update counters
    if ready
        if row_counter < max_row_count 
            row_counter(:) = row_counter + 1; 
        else          
            
            if col_counter < m_cols
                row_counter(:) = 1;
                col_counter(:) = col_counter + 1; % next column
            else
                if waitForDone %wait for done
                    row_counter(:) = 1;
                    col_counter(:) = 1; % reset to beginning of matrix
                    stop_write = false; % set to true to stop indefinite reads
                else
                    stop_write = true;
                end
            end
        end
    else
        valid_out = false;
    end

end

== matlab function ddrxpose_21a_generic/XDF/FromDDRMemory1/videoTimingGenerator ==
  data: start input boolean; ctrlO output Bus: pixelcontrol; hBlank parameter; vBlank parameter; hSize parameter; vSize parameter; delayStartClks parameter
function ctrlO  = ctrlGenerator(start, hBlank, vBlank, hSize, vSize, delayStartClks)

%% define states used
IDLE             = fi(0,0,3,0);
DELAYSTART       = fi(1,0,3,0);
ACTIVELINE       = fi(3,0,3,0);
ACTIVELINEBLANK  = fi(7,0,3,0);
ACTIVEFRAMEBLANK = fi(4,0,3,0);

%% persistent variables declared here
persistent state hPos vPos ...
           valid hStart vStart hEnd vEnd ...
           blankCnt startDelayCnt
       
if isempty(state)
    state = IDLE;
    hPos = uint32(0);
    vPos = uint32(0);
    valid = false;
    hStart = false;
    vStart = false;
    hEnd = false;
    vEnd = false;
    blankCnt = uint32(0);
    startDelayCnt = uint32(0);
 end

%% output the states of the FSM here
ctrlO = struct('hStart', hStart, 'hEnd', hEnd, 'vStart', vStart, 'vEnd', vEnd, 'valid', valid);


%% FSM for streaming out the frame
switch state
    case IDLE
        % wait for the start trigger
        if start
            state = DELAYSTART;
            startDelayCnt(:) = 0;
        end
    case DELAYSTART
        startDelayCnt(:) = startDelayCnt + 1;
        if startDelayCnt == delayStartClks
            hStart = true;
            vStart = true;
            hEnd = false;
            vEnd = false;
            valid = true;
            state = ACTIVELINE;
            vPos(:) = 1;
            hPos(:) = 1;
        end
    case ACTIVELINE
    % active line pixels
        hStart = false;
        vStart = false;
        valid = true;
        hPos(:) = hPos + 1;
        if hPos == hSize
            state = ACTIVELINEBLANK;
            hEnd = true;
            blankCnt(:) = 0;
            if vPos == vSize
                vEnd = true;
                state = ACTIVEFRAMEBLANK;
            end
        end
    case ACTIVELINEBLANK
    % end of the active line output - Active Horz Blanking
        hEnd = false;        
        valid = false;
        blankCnt(:) = blankCnt + 1;
        if blankCnt == hBlank
            hPos(:) = 1;
            vPos(:) = vPos + 1;
            state = ACTIVELINE;
            hStart = true;
            valid = true;
        end
    case ACTIVEFRAMEBLANK
        %  end of active frame - Active Vert Blanking
        hEnd = false;        
        vEnd = false;
        valid = false;
        blankCnt(:) = blankCnt + 1;
        if blankCnt == (vBlank * hSize)
            state = IDLE;
        end
end
